simulink model "example4"  (R2022b)
settings: Solver=FixedStepDiscrete  StartTime=0.0  StopTime=Tges  RelTol=1e-3
model workspace (MAT data in the model file):
  Tges = 500000
  Ts = 5
settings Model: Creator=siegl  LastModifiedBy=chris
settings DebuggingCC: UnconnectedInputMsg=warning  UnconnectedOutputMsg=warning  UnconnectedLineMsg=warning
settings ModelReferenceCC: EnableRefExpFcnMdlSchedulingChecks=on
settings RTWCC: DLArmComputeVersion=19.05

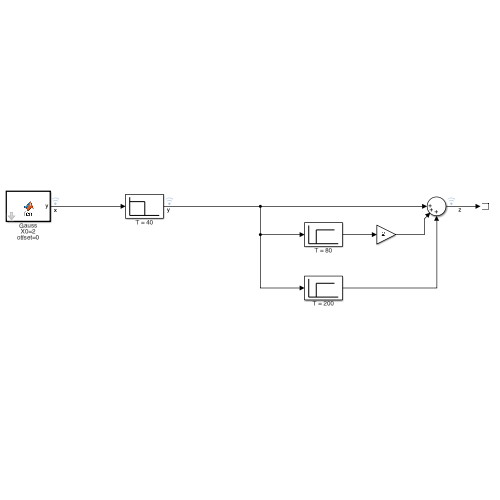
[thumbnail: Simulink's stored preview of the top-level diagram]
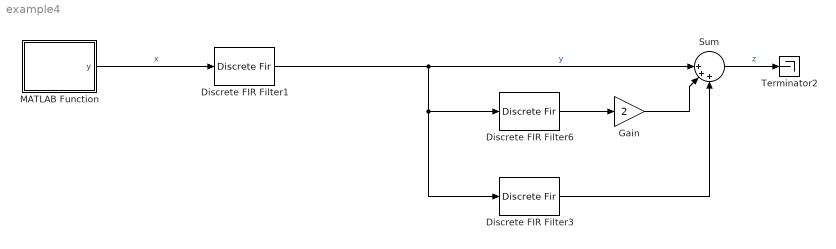
== system example4 ==
  Discrete FIR Filter1 : DiscreteFir  Coefficients=ones(1,Tavg/SampleTime)*SampleTime/Tavg  SampleTime=SampleTime  mask{Tavg=40, SampleTime=Ts}
      mask prompts: Tavg "Average Time"; SampleTime "Simulink:blkprm_prompts:AllBlksSampleTime"
      settings: AttributesFormatString=T = %<Tavg>
      mask TypeOptions SampleTime: SampleTime
      mask DialogControl SampleTime Prompt: Sample time (-1 for inherited):
      mask Display:
      | plot([0.1, .9], [.1, .1])
      | plot([0.1, .1], [.1, .9])
      | plot([0.1, .5], [.7, .7])
      | plot([0.5, .5], [.7, .1])
  Discrete FIR Filter3 : DiscreteFir  Coefficients=[zeros(1,Td/SampleTime), 1]  SampleTime=SampleTime  mask{Td=200, SampleTime=Ts}
      mask prompts: Td "Delay Time"; SampleTime "Simulink:blkprm_prompts:AllBlksSampleTime"
      settings: AttributesFormatString=T = %<Td>
      mask TypeOptions SampleTime: SampleTime
      mask DialogControl SampleTime Prompt: Sample time (-1 for inherited):
      mask Display:
      | plot([0.1, .9], [.1, .1])
      | plot([0.1, .1], [.1, .9])
      | plot([0.3, .3], [.7, .1])
      | plot([0.3, .8], [.7, .7])
  Discrete FIR Filter6 : DiscreteFir  Coefficients=[zeros(1,Td/SampleTime), 1]  SampleTime=SampleTime  mask{Td=80, SampleTime=Ts}
      mask prompts: Td "Delay Time"; SampleTime "Simulink:blkprm_prompts:AllBlksSampleTime"
      settings: AttributesFormatString=T = %<Td>
      mask TypeOptions SampleTime: SampleTime
      mask DialogControl SampleTime Prompt: Sample time (-1 for inherited):
      mask Display:
      | plot([0.1, .9], [.1, .1])
      | plot([0.1, .1], [.1, .9])
      | plot([0.3, .3], [.7, .1])
      | plot([0.3, .8], [.7, .7])
  Gain : Gain  Gain=2
  MATLAB Function : MATLAB Function  TreatAsAtomicUnit=on  mask{mu=0, sigma2=2, distribution=Gauss, T=Ts}
      mask prompts: mu "Mean"; sigma2 "Variance"; T "Sample Time"
      settings: AttributesFormatString=|
      | %<distribution>
      | X0=%<sigma2>
      | offset=%<mu>
  Sum : Sum  Inputs=||+++
  Terminator2 : Terminator
  wires:
  Sum/1 -> Terminator2/1  "z"
  MATLAB Function/1(y) -> Discrete FIR Filter1/1  "x"
  Discrete FIR Filter1/1 -> Sum/1, Discrete FIR Filter3/1, Discrete FIR Filter6/1  "y"
  Discrete FIR Filter6/1 -> Gain/1
  Discrete FIR Filter3/1 -> Sum/3
  Gain/1 -> Sum/2

== matlab function example4/MATLAB Function ==
  data: y output; mu parameter; sigma2 parameter; T parameter; distribution parameter
function y = fcn(mu, sigma2, T, distribution)

if distribution == 1
    X = (sqrt(12)*(rand(1,1)-0.5));
else
    X = randn(1,1);
end

y = sqrt(sigma2/T)*X+mu;
